simulink model "sampleModel1901"  (R2023a)
settings: Solver=VariableStepAuto  StartTime=0.0  StopTime=10.0  RelTol=1e-3
libraries: hdlsllib x8
settings Model: Creator=user1  LastModifiedBy=user1

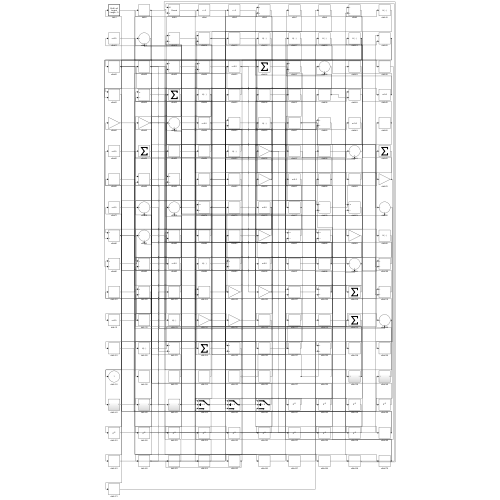
[thumbnail: Simulink's stored preview of the top-level diagram]
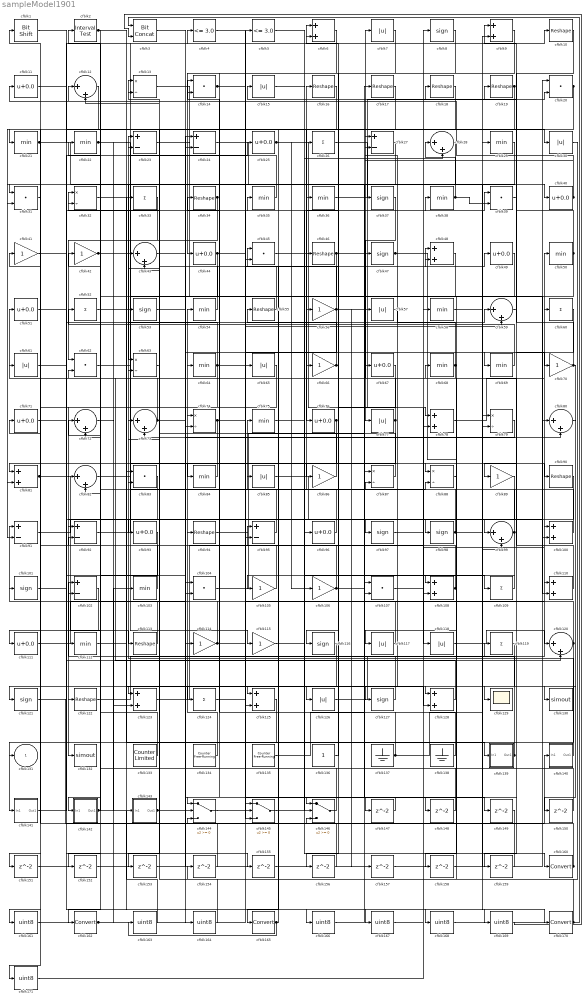
== system sampleModel1901 ==
  cfblk1 : hdlsllib/Logic and Bit Operations/Bit Shift  mode=Shift Left Logical  N=0
  cfblk{10,16..19,34,46,55,90,94,113,122} (12 alike) : Reshape
  cfblk{6,9,48,78,81,100,108,110,123,125,128} (11 alike) : Sum
  cfblk{8,37,47,53,97..98,101,116,121,127} (10 alike) : Signum
  cfblk{23..24,27,91..92,95,102} (7 alike) : Sum  Inputs=+-
  cfblk{21..22,29,35..36,38,50,54,58,64,68..69,75,84,103,112} (16 alike) : MinMax
  cfblk{14,20,31,39,45,62,83,104,107} (9 alike) : DotProduct  OutDataTypeStr=Inherit: Inherit via internal rule
  cfblk{41..42,56,66,70,86,89,105..106,114..115} (11 alike) : Gain
  cfblk{26,33,52,60,109,119,124} (7 alike) : Sum  Inputs=+
  cfblk{11,25,40,44,49,51,67,71,76,93,96,111} (12 alike) : Bias  Bias=0.0  SaturateOnIntegerOverflow=off
  cfblk{7,15,30,57,61,65,77,85,117..118,126} (11 alike) : Abs  SaturateOnIntegerOverflow=off
  cfblk{12,28,43,59,72..73,80,82,99,120} (10 alike) : Sum  Inputs=|++
  cfblk129 : Scope
  cfblk{13,32,63,74,79,87..88} (7 alike) : Product  Inputs=*/  RndMeth=Zero  SaturateOnIntegerOverflow=on
  cfblk130 : ToWorkspace  VariableName=simout  SaveFormat=Timeseries  SampleTime=-1
  cfblk132 : ToWorkspace  VariableName=simout  SaveFormat=Timeseries  SampleTime=-1
  cfblk133 : hdlsllib/Sources/Counter Limited  uplimit=7  tsamp=-1
  cfblk134 : hdlsllib/Sources/Counter Free-Running  NumBits=16  tsamp=-1
  cfblk135 : hdlsllib/Sources/Counter Free-Running  NumBits=16  tsamp=-1
  cfblk136 : Constant  SampleTime=-1
  cfblk137 : Ground
  cfblk138 : Ground
  cfblk139 : Subsystem
      settings: LibrarySourceBlock=|
      | hdlsllib/Ports &
      | Subsystems/Subsystem
  cfblk140 : Subsystem
      settings: LibrarySourceBlock=|
      | hdlsllib/Ports &
      | Subsystems/Subsystem
  cfblk141 : Subsystem
      settings: LibrarySourceBlock=|
      | hdlsllib/Ports &
      | Subsystems/Subsystem
  cfblk142 : Subsystem
      settings: LibrarySourceBlock=|
      | hdlsllib/Ports &
      | Subsystems/Subsystem
  cfblk143 : Subsystem
      settings: LibrarySourceBlock=|
      | hdlsllib/Ports &
      | Subsystems/Subsystem
  cfblk144 : Switch  SaturateOnIntegerOverflow=off  InputSameDT=off
  cfblk145 : Switch  SaturateOnIntegerOverflow=off  InputSameDT=off
  cfblk146 : Switch  SaturateOnIntegerOverflow=off  InputSameDT=off
  cfblk{147..159} (13 alike) : Delay  SampleTime=1
  cfblk{160,162,165,170} (4 alike) : DataTypeConversion  SaturateOnIntegerOverflow=off  RndMeth=Floor
  cfblk{161,163..164,166..169,171} (8 alike) : DataTypeConversion  OutDataTypeStr=uint8  SaturateOnIntegerOverflow=off  RndMeth=Floor
  cfblk2 : hdlsllib/Logic and Bit Operations/Interval Test  IntervalClosedRight=on  uplimit=0.5  IntervalClosedLeft=on  lowlimit=-0.5  OutDataTypeStr=boolean
  cfblk3 : hdlsllib/Logic and Bit Operations/Bit Concat  numInputs=2
  cfblk4 : hdlsllib/Logic and Bit Operations/Compare To Constant  relop=<=  const=3.0  OutDataTypeStr=boolean
  cfblk5 : hdlsllib/Logic and Bit Operations/Compare To Constant  relop=<=  const=3.0  OutDataTypeStr=boolean
  cfblk131 : Outport  VectorParamsAs1DForOutWhenUnconnected=off
  wires:
  cfblk40/1 -> cfblk12/1, cfblk27/2
  cfblk98/1 -> cfblk16/1, cfblk6/1, cfblk99/2
  cfblk72/1 -> cfblk143/1(In1)
  cfblk139/1(Out1) -> cfblk54/1, cfblk34/1
  cfblk42/1 -> cfblk88/1, cfblk139/1(In1)
  cfblk18/1 -> cfblk76/1
  cfblk37/1 -> cfblk77/1
  cfblk47/1 -> cfblk117/1, cfblk110/2
  cfblk52/1 -> cfblk115/1
  cfblk77/1 -> cfblk7/1, cfblk112/1
  cfblk34/1 -> cfblk62/1, cfblk74/2
  cfblk38/1 -> cfblk28/1, cfblk39/2
  cfblk25/1 -> cfblk69/1, cfblk106/1
  cfblk39/1 -> cfblk146/1
  cfblk26/1 -> cfblk78/1
  cfblk109/1 -> cfblk108/1
  cfblk128/1 -> cfblk51/1
  cfblk62/1 -> cfblk35/1
  cfblk60/1 -> cfblk89/1
  cfblk76/1 -> cfblk125/1, cfblk95/2
  cfblk92/1 -> cfblk4/1
  cfblk5/1 -> cfblk160/1
  cfblk140/1(Out1) -> cfblk23/1
  cfblk105/1 -> cfblk64/1
  cfblk4/1 -> cfblk145/1
  cfblk24/1 -> cfblk87/1
  cfblk85/1 -> cfblk98/1
  cfblk81/1 -> cfblk113/1, cfblk168/1
  cfblk65/1 -> cfblk132/1
  cfblk27/1 -> cfblk63/1
  cfblk86/1 -> cfblk32/1
  cfblk13/1 -> cfblk40/1
  cfblk54/1 -> cfblk11/1
  cfblk79/1 -> cfblk73/2
  cfblk114/1 -> cfblk126/1, cfblk101/1
  cfblk2/1 -> cfblk142/1(In1), cfblk100/2
  cfblk134/1 -> cfblk94/1
  cfblk32/1 -> cfblk57/1
  cfblk6/1 -> cfblk145/2
  cfblk83/1 -> cfblk162/1
  cfblk91/1 -> cfblk93/1
  cfblk50/1 -> cfblk128/1, cfblk19/1
  cfblk75/1 -> cfblk109/1
  cfblk123/1 -> cfblk78/2
  cfblk9/1 -> cfblk26/1
  cfblk78/1 -> cfblk50/1
  cfblk15/1 -> cfblk28/2
  cfblk136/1 -> cfblk36/1
  cfblk145/1 -> cfblk96/1
  cfblk87/1 -> cfblk53/1
  cfblk46/1 -> cfblk84/1, cfblk149/1
  cfblk17/1 -> cfblk165/1
  cfblk122/1 -> cfblk60/1
  cfblk67/1 -> cfblk86/1
  cfblk127/1 -> cfblk102/1
  cfblk69/1 -> cfblk52/1
  cfblk64/1 -> cfblk81/1, cfblk10/1, cfblk59/2, cfblk43/2
  cfblk35/1 -> cfblk13/1
  cfblk110/1 -> cfblk62/2
  cfblk121/1 -> cfblk140/1(In1)
  cfblk117/1 -> cfblk2/1
  cfblk23/1 -> cfblk80/1
  cfblk20/1 -> cfblk21/1, cfblk123/1
  cfblk36/1 -> cfblk18/1
  cfblk138/1 -> cfblk74/1
  cfblk125/1 -> cfblk141/1(In1)
  cfblk70/1 -> cfblk130/1, cfblk15/1
  cfblk84/1 -> cfblk82/1
  cfblk19/1 -> cfblk116/1, cfblk91/2, cfblk111/1
  cfblk90/1 -> cfblk122/1
  cfblk124/1 -> cfblk110/1
  cfblk115/1 -> cfblk38/1
  cfblk66/1 -> cfblk55/1, cfblk46/1
  cfblk118/1 -> cfblk120/1
  cfblk7/1 -> cfblk144/1
  cfblk144/1 -> cfblk59/1
  cfblk61/1 -> cfblk97/1
  cfblk97/1 -> cfblk20/2
  cfblk45/1 -> cfblk118/1
  cfblk68/1 -> cfblk63/2, cfblk27/1
  cfblk82/1 -> cfblk88/2
  cfblk58/1 -> cfblk170/1
  cfblk8/1 -> cfblk44/1
  cfblk100/1 -> cfblk75/1
  cfblk119/1 -> cfblk121/1
  cfblk44/1 -> cfblk99/1, cfblk153/1
  cfblk143/1(Out1) -> cfblk80/2, cfblk43/1
  cfblk108/1 -> cfblk61/1, cfblk105/1
  cfblk126/1 -> cfblk119/1
  cfblk33/1 -> cfblk92/1
  cfblk51/1 -> cfblk120/2
  cfblk113/1 -> cfblk91/1
  cfblk73/1 -> cfblk37/1, cfblk22/1
  cfblk94/1 -> cfblk87/2
  cfblk14/1 -> cfblk65/1, cfblk147/1
  cfblk142/1(Out1) -> cfblk92/2, cfblk166/1
  cfblk56/1 -> cfblk12/2, cfblk90/1, cfblk125/2, cfblk157/1
  cfblk29/1 -> cfblk124/1
  cfblk74/1 -> cfblk49/1, cfblk48/1, cfblk161/1
  cfblk95/1 -> cfblk72/1
  cfblk111/1 -> cfblk24/2
  cfblk49/1 -> cfblk82/2
  cfblk96/1 -> cfblk13/2
  cfblk22/1 -> cfblk114/1, cfblk128/2, cfblk123/2
  cfblk106/1 -> cfblk45/1, cfblk48/2
  cfblk133/1 -> cfblk72/2
  cfblk103/1 -> cfblk41/1
  cfblk99/1 -> cfblk42/1, cfblk158/1
  cfblk104/1 -> cfblk67/1
  cfblk48/1 -> cfblk146/2
  cfblk137/1 -> cfblk14/1, cfblk29/1
  cfblk16/1 -> cfblk31/1
  cfblk53/1 -> cfblk70/1
  cfblk12/1 -> cfblk31/2
  cfblk63/1 -> cfblk23/2
  cfblk57/1 -> cfblk127/1
  cfblk28/1 -> cfblk81/2
  cfblk101/1 -> cfblk25/1
  cfblk112/1 -> cfblk33/1
  cfblk107/1 -> cfblk100/1
  cfblk59/1 -> cfblk9/1
  cfblk55/1 -> cfblk14/2
  cfblk1/1 -> cfblk104/2
  cfblk31/1 -> cfblk131/1
  cfblk120/1 -> cfblk66/1, cfblk129/1, cfblk145/3
  cfblk141/1(Out1) -> cfblk39/1
  cfblk21/1 -> cfblk79/1, cfblk6/2, cfblk169/1
  cfblk135/1 -> cfblk47/1
  cfblk146/1 -> cfblk95/1
  cfblk11/1 -> cfblk30/1
  cfblk71/1 -> cfblk56/1
  cfblk147/1 -> cfblk144/2
  cfblk88/1 -> cfblk148/1
  cfblk148/1 -> cfblk32/2
  cfblk149/1 -> cfblk144/3
  cfblk80/1 -> cfblk150/1
  cfblk150/1 -> cfblk102/2
  cfblk116/1 -> cfblk151/1
  cfblk151/1 -> cfblk104/1
  cfblk93/1 -> cfblk152/1
  cfblk152/1 -> cfblk9/2
  cfblk153/1 -> cfblk107/2
  cfblk30/1 -> cfblk154/1
  cfblk154/1 -> cfblk73/1
  cfblk41/1 -> cfblk155/1
  cfblk155/1 -> cfblk20/1
  cfblk89/1 -> cfblk156/1
  cfblk156/1 -> cfblk24/1
  cfblk157/1 -> cfblk108/2
  cfblk158/1 -> cfblk79/2
  cfblk10/1 -> cfblk159/1
  cfblk159/1 -> cfblk1/1
  cfblk160/1 -> cfblk146/3, cfblk71/1
  cfblk161/1 -> cfblk5/1
  cfblk162/1 -> cfblk45/2, cfblk103/1
  cfblk163/1 -> cfblk83/1
  cfblk43/1 -> cfblk164/1
  cfblk164/1 -> cfblk83/2
  cfblk165/1 -> cfblk163/1, cfblk85/1
  cfblk166/1 -> cfblk17/1
  cfblk3/1 -> cfblk167/1
  cfblk167/1 -> cfblk8/1
  cfblk168/1 -> cfblk3/1
  cfblk169/1 -> cfblk3/2
  cfblk170/1 -> cfblk68/1, cfblk107/1
  cfblk102/1 -> cfblk171/1
  cfblk171/1 -> cfblk58/1

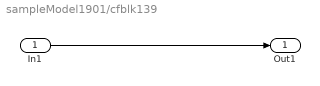
== system sampleModel1901/cfblk139 ==
  In1 : Inport
  Out1 : Outport
  wires:
  In1/1 -> Out1/1

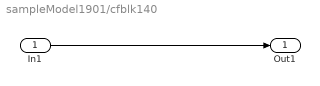
== system sampleModel1901/cfblk140 ==
  In1 : Inport
  Out1 : Outport
  wires:
  In1/1 -> Out1/1

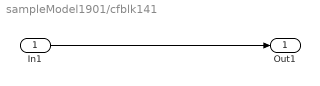
== system sampleModel1901/cfblk141 ==
  In1 : Inport
  Out1 : Outport
  wires:
  In1/1 -> Out1/1

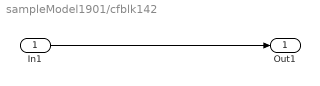
== system sampleModel1901/cfblk142 ==
  In1 : Inport
  Out1 : Outport
  wires:
  In1/1 -> Out1/1

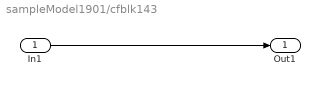
== system sampleModel1901/cfblk143 ==
  In1 : Inport
  Out1 : Outport
  wires:
  In1/1 -> Out1/1
